simulink model "extTorqueObserver"  (R2018a)
settings: Solver=VariableStepAuto  StartTime=0.0  StopTime=10.0  RelTol=1e-3
values from neighbouring files (symbols this model uses):
  D = 0.01    [torqueObserverData.m]
  Denv = 1    [torqueObserverData.m]
  F = 0.01    [torqueObserverData.m]
  g_reac = 500    [torqueObserverData.m]
  J = 0.1    [torqueObserverData.m]
  Jn = 0.1    [torqueObserverData.m]
  Kenv = 2    [torqueObserverData.m]
  Kt = 1    [torqueObserverData.m]
  Ktn = 0.1    [torqueObserverData.m]
  L = 1    [torqueObserverData.m]
  M = 1    [torqueObserverData.m]
libraries: simulink x1
settings Model: Creator=dinies33  LastModifiedBy=blue_orangotan

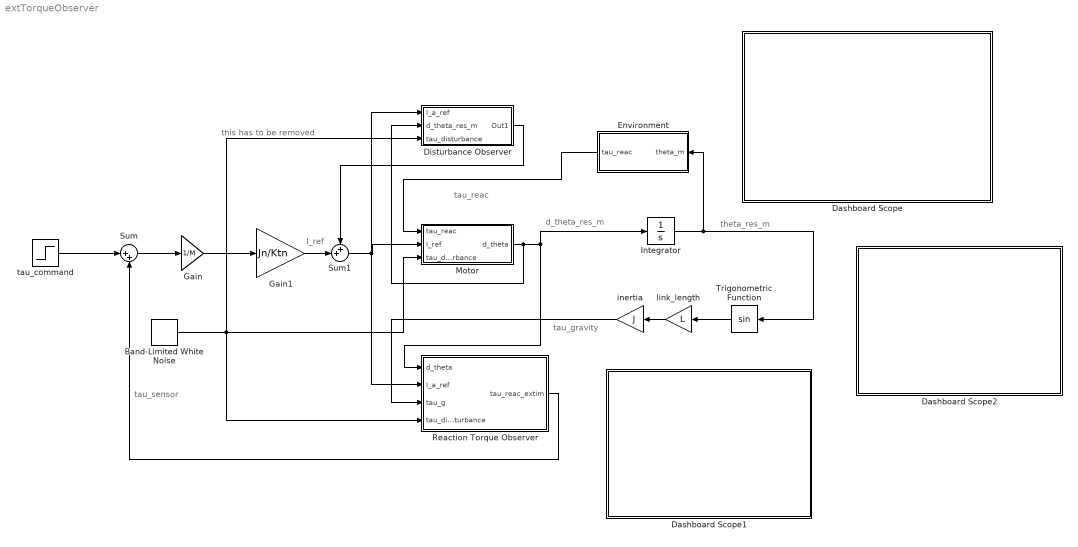
== system extTorqueObserver ==
  note: tau_gravity
  note: this has to be removed
  note: tau_sensor
  note: tau_reac
  note: theta_res_m
  note: d_theta_res_m
  note: I_ref
  Band-Limited White Noise : simulink/Sources/Band-Limited White Noise  Cov=0.01  Ts=0.1  seed=[23341]
  Dashboard Scope : Subsystem  DialogController=hmiCreateDDGDialog  IsWebBlock=on  mask(MWDashboardBlock){webBlockId=e89d37ff-74b8-4979-92f7-4f92c8cfe862, webBlockType=sdiscope, ShowInitialText=on, HMISrcModelName=extTorqueObserver}
      mask prompts: webBlockId "WebBlock Id"; webBlockType "WebBlock Type"; HMISrcModelName "Source Model"
      mask help: SimulinkHMI:dialogs:HMIScopeDialogDesc
      mask Help: helpview([docroot '/mapfiles/simulink.map'], 'hmi_scope')
      mask Display:
      | if strcmp(get_param(bdroot(gcb),'BlockDiagramType'), 'library')
      |     image([(matlabroot) '/toolbox/simulink/hmi/icons/DashboardScope.png']);
      | end
  Dashboard Scope1 : Subsystem  DialogController=hmiCreateDDGDialog  IsWebBlock=on  mask(MWDashboardBlock){webBlockId=b0ee7d7c-c0a2-4845-8648-566948305a11, webBlockType=sdiscope, ShowInitialText=on, HMISrcModelName=extTorqueObserver}
      mask prompts: webBlockId "WebBlock Id"; webBlockType "WebBlock Type"; HMISrcModelName "Source Model"
      mask help: SimulinkHMI:dialogs:HMIScopeDialogDesc
      mask Help: helpview([docroot '/mapfiles/simulink.map'], 'hmi_scope')
      mask Display:
      | if strcmp(get_param(bdroot(gcb),'BlockDiagramType'), 'library')
      |     image([(matlabroot) '/toolbox/simulink/hmi/icons/DashboardScope.png']);
      | end
  Dashboard Scope2 : Subsystem  DialogController=hmiCreateDDGDialog  IsWebBlock=on  mask(MWDashboardBlock){webBlockId=3fbafb71-391f-42f7-a6aa-5462446d1dbe, webBlockType=sdiscope, ShowInitialText=on, HMISrcModelName=extTorqueObserver}
      mask prompts: webBlockId "WebBlock Id"; webBlockType "WebBlock Type"; HMISrcModelName "Source Model"
      mask help: SimulinkHMI:dialogs:HMIScopeDialogDesc
      mask Help: helpview([docroot '/mapfiles/simulink.map'], 'hmi_scope')
      mask Display:
      | if strcmp(get_param(bdroot(gcb),'BlockDiagramType'), 'library')
      |     image([(matlabroot) '/toolbox/simulink/hmi/icons/DashboardScope.png']);
      | end
  Disturbance Observer : Subsystem
  Environment : Subsystem
  Gain : Gain  Gain=1/M
  Gain1 : Gain  Gain=Jn/Ktn
  Integrator : Integrator
  Motor : Subsystem
  "Reaction Torque Observer " : Subsystem
  Sum : Sum  Inputs=|++
  Sum1 : Sum  Inputs=++|
  Trigonometric Function : Trigonometry
  "inertia " : Gain  Gain=J
  "link_length " : Gain  Gain=L
  tau_command : Step  After=5  SampleTime=0
  wires:
  Sum/1 -> Gain/1
  Gain/1 -> Gain1/1
  Sum1/1 -> Disturbance Observer/1("I_a_ref "), Motor/2(I_ref), "Reaction Torque Observer "/2("I_a_ref ")
  Motor/1("d_theta ") -> "Reaction Torque Observer "/1("d_theta "), Integrator/1, Disturbance Observer/2("d_theta_res_m ")
  "Reaction Torque Observer "/1("tau_reac_extim ") -> Sum/2
  Environment/1("tau_reac ") -> Motor/1(tau_reac)
  Integrator/1 -> Trigonometric Function/1, Environment/1(theta_m)
  tau_command/1 -> Sum/1
  Gain1/1 -> Sum1/2
  Disturbance Observer/1(Out1) -> Sum1/1
  Band-Limited White Noise/1 -> "Reaction Torque Observer "/4("tau_disturbance "), Disturbance Observer/3("tau_disturbance "), Motor/3("tau_disturbance ")
  "link_length "/1 -> "inertia "/1
  "inertia "/1 -> "Reaction Torque Observer "/3("tau_g ")
  Trigonometric Function/1 -> "link_length "/1

== system extTorqueObserver/Dashboard Scope ==

== system extTorqueObserver/Dashboard Scope1 ==

== system extTorqueObserver/Dashboard Scope2 ==

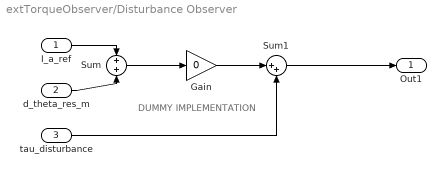
== system extTorqueObserver/Disturbance Observer ==
  note: DUMMY IMPLEMENTATION
  "I_a_ref " : Inport
  "d_theta_res_m " : Inport  Port=2
  "tau_disturbance " : Inport  Port=3
  Gain : Gain  Gain=0
  Sum : Sum  Inputs=+|+
  Sum1 : Sum  Inputs=|++
  Out1 : Outport
  wires:
  "I_a_ref "/1 -> Sum/1
  "d_theta_res_m "/1 -> Sum/2
  Sum/1 -> Gain/1
  Gain/1 -> Sum1/1
  "tau_disturbance "/1 -> Sum1/2
  Sum1/1 -> Out1/1

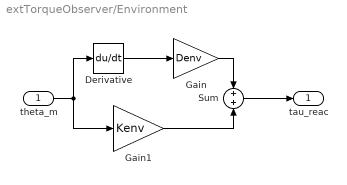
== system extTorqueObserver/Environment ==
  theta_m : Inport
  Derivative : Derivative  CoefficientInTFapproximation=1
  Gain : Gain  Gain=Denv
  Gain1 : Gain  Gain=Kenv
  Sum : Sum  Inputs=+|+
  "tau_reac " : Outport
  wires:
  Derivative/1 -> Gain/1
  Gain/1 -> Sum/1
  Sum/1 -> "tau_reac "/1
  theta_m/1 -> Gain1/1, Derivative/1
  Gain1/1 -> Sum/2

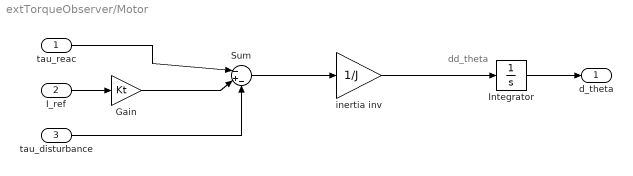
== system extTorqueObserver/Motor ==
  note: dd_theta
  tau_reac : Inport
  I_ref : Inport  Port=2
  "tau_disturbance " : Inport  Port=3
  Gain : Gain  Gain=Kt
  Integrator : Integrator
  Sum : Sum  Inputs=|-+-
  "inertia inv " : Gain  Gain=1/J
  "d_theta " : Outport
  wires:
  Gain/1 -> Sum/2
  Sum/1 -> "inertia inv "/1
  I_ref/1 -> Gain/1
  tau_reac/1 -> Sum/1
  "inertia inv "/1 -> Integrator/1
  Integrator/1 -> "d_theta "/1
  "tau_disturbance "/1 -> Sum/3

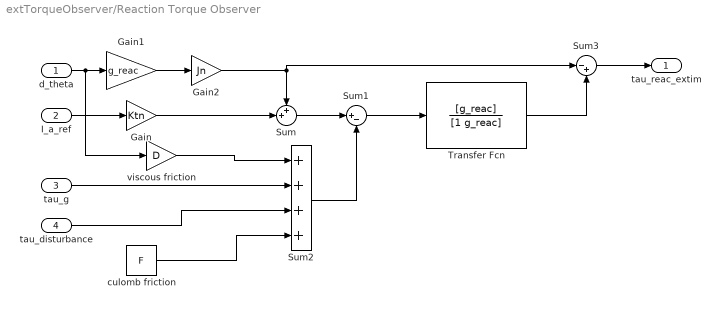
== system extTorqueObserver/Reaction Torque Observer  ==
  "d_theta " : Inport
  "I_a_ref " : Inport  Port=2
  "tau_g " : Inport  Port=3
  "tau_disturbance " : Inport  Port=4
  Gain : Gain  Gain=Ktn
  Gain1 : Gain  Gain=g_reac
  Gain2 : Gain  Gain=Jn
  Sum : Sum  Inputs=++|
  Sum1 : Sum  Inputs=|+-
  Sum2 : Sum  Inputs=++++
  Sum3 : Sum  Inputs=|-+
  Transfer Fcn : TransferFcn  Numerator=[g_reac]  Denominator=[1 g_reac]
  "culomb friction " : Constant  Value=F
  "viscous friction " : Gain  Gain=D
  "tau_reac_extim " : Outport
  wires:
  "I_a_ref "/1 -> Gain/1
  "d_theta "/1 -> "viscous friction "/1, Gain1/1
  Gain1/1 -> Gain2/1
  Gain/1 -> Sum/2
  Gain2/1 -> Sum3/1, Sum/1
  Sum/1 -> Sum1/1
  Sum2/1 -> Sum1/2
  "viscous friction "/1 -> Sum2/1
  "culomb friction "/1 -> Sum2/4
  Sum3/1 -> "tau_reac_extim "/1
  Sum1/1 -> Transfer Fcn/1
  Transfer Fcn/1 -> Sum3/2
  "tau_g "/1 -> Sum2/2
  "tau_disturbance "/1 -> Sum2/3
